simulink model "A"  (R2022b)
settings: Solver=VariableStepAuto  StartTime=0.0  StopTime=10.0  RelTol=1e-3
settings Model: DataDictionary=A.sldd  Creator=LYZ  LastModifiedBy=LYZ

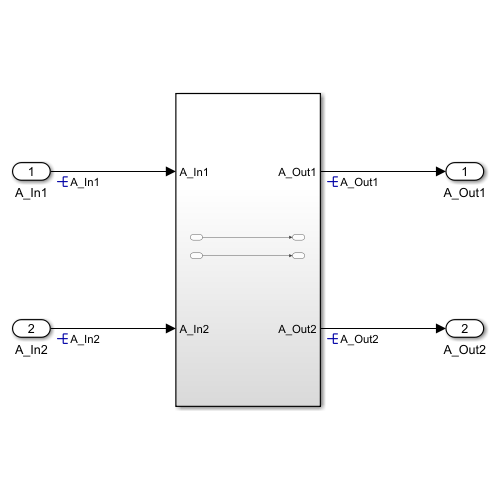
[thumbnail: Simulink's stored preview of the top-level diagram]
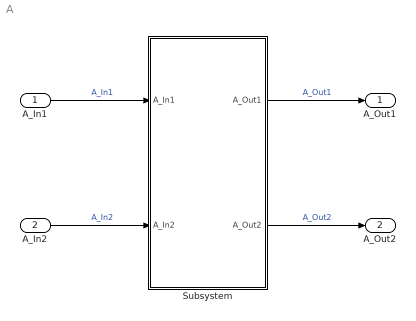
== system A ==
  A_In1 : Inport
  A_In2 : Inport  Port=2
  Subsystem : Subsystem
  A_Out1 : Outport
  A_Out2 : Outport  Port=2
  wires:
  A_In1/1 -> Subsystem/1(A_In1)  "A_In1"
  A_In2/1 -> Subsystem/2(A_In2)  "A_In2"
  Subsystem/1(A_Out1) -> A_Out1/1  "A_Out1"
  Subsystem/2(A_Out2) -> A_Out2/1  "A_Out2"

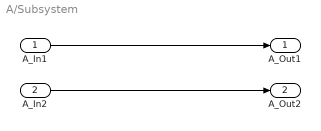
== system A/Subsystem ==
  A_In1 : Inport
  A_In2 : Inport  Port=2
  A_Out1 : Outport
  A_Out2 : Outport  Port=2
  wires:
  A_In1/1 -> A_Out1/1
  A_In2/1 -> A_Out2/1
